simulink model "EKF_sim"  (R2020a)
settings: Solver=VariableStepAuto  StartTime=0.0  StopTime=694  RelTol=1e-3
values from neighbouring files (symbols this model uses):
  acc_variance = 4.8e-1    (= 0.48)    [init.m]
  bias_acc_variance = 4e-10    [init.m]
  bias_gyro_variance = 4e-14    [init.m]
  DT = EKF_DT    (= 0.02)    [init.m]
  EKF_DT = 0.02    [init.m]
  g = 9.81    [init.m]
  GPS_variance = 1e-2    (= 0.01)    [init.m]
  gyro_variance = 4.8e-2    (= 0.048)    [init.m]
  head_variance = 7e-3    (= 0.007)    [init.m]
  init_time = 11    [init.m]
  lambda_xa = 1e-4    (= 0.0001)    [init.m]
  lambda_xg = 1e-3    (= 0.001)    [init.m]
  SHOE_buffer_N = 100    [init.m]
  SHOE_threshold = 30    [init.m]
  t1_end = 291    [init.m]
  t1_start = 290    [init.m]
  t2_end = 392.5    [init.m]
  t2_start = 392    [init.m]
  t3_end = 420    [init.m]
  t3_start = 419    [init.m]
  t4_end = 439    [init.m]
  t4_start = 438    [init.m]
  vel_variance = 1e-2    (= 0.01)    [init.m]
  zero_vel_period = 50000    [init.m]
(part 4 of 5)

== matlab function EKF_sim/EKF_bias/System Prediction/prediction_step ==
  data: x0 input; x_k output; P0 input; x_k_1 input size=22 1; P_k_1 input size=22 22; yg input; ya input; lambda_xa parameter; lambda_xg parameter; U input; P_k output size=22 22; DT parameter; g parameter; flag_init input; flag_init_ output
% --------------------         prediction           -------------------- %
%{
% This function computes the prediction step of the Kalman Filter. After 
% the initialization of the system, at each period the state vector is 
% updated, related to the prediction function and the measurement by the 
% inertial sensors (gyroscope and accelerometer). The covariance matrix P 
% is also updated.

% Input:
%     x0         : initial vector state
%     P0         : initial matrix P
%     x_k_1      : state vector before prediction step
%     P_k_1      : matrix P before prediction step
%     yg         : gyroscope measurement
%     ya         : accelerometer measurement
%     lambda_xa  : correlation time of Accelerometer Bias
%     lambda_xg  : correlation time of Gyroscope Bias
%     U          : covariance Matrix of input sensor
%     DT         : period of EKF system
%     g          : gravity acceleration
%     flag_init  : flag for initialization task

% Output:
%     x_k        : state vector after prediction step
%     P_k        : matrix P after prediction step
%     flag_init_ : flag for initialization task

% State vector x = [q w xg r v a xa]' [22x1]:
% q  = [q1 q2 q3 q4]     unit quaternion representing the attitude (1 2 3 4)
% w  = [wx wy wz]        angular velocity (5 6 7)
% xg = [xg_x xg_y xg_z]  gyro bias (8 9 10)
% r  = [rx ry rz]        position (NED)(11 12 13)
% v  = [vx vy vz]        linear velocity (NED) (14 15 16)
% a  = [ax ay az]        linear acceleration (NED) (17 18 19)
% xa = [xa_x xa_y xa_z]  accelerometer bias (20 21 22)
 
% Prediction model functions:
% fq = q * q(w*DT)
% fw = (yg-xg);
% fxg = (1-lambda_xg*DT)*xg+vxg;
% fr = r + v*DT + a*DT*DT/2;
% fv = v + a*DT;
% fa = Rnb*(ya - xa) + [0;0;g];
% fxa = (1-lambda_xa*DT)*xa+vxa;

% P_k = Fx*P_k_1*Fx' + Fu*U*Fu'
 
% U = [gyro_variance(3x3),       0               0               0
%        0           bias_gyro_variance(3x3)     0               0
%        0                       0        acc_variance(3x3)      0
%        0                       0                  bias_acc_variance(3x3)]

% See 'calcolo_matrice_F.m' for the exact calculation of matrices Fx and Fu
% These matrices are calculated offline, so note that if same parameters of 
% the system change, these matrices need to be changed.
%}
%%
function [x_k,  P_k, flag_init_] = prediction(x0, P0, x_k_1, P_k_1, ...
                                          yg, ya, lambda_xa, lambda_xg,...
                                          U, DT, g, flag_init)
    x_k = zeros(22,1);
    P_k = zeros(22,22);
    flag_init_ = flag_init;
    if flag_init ~= 0           %initialization check
        if flag_init == 1
            x_k_1 = x0;
            P_k_1 = P0;
            flag_init_ = 2;     %set flag=2 so the initialization is done
        end                     %one time only
        
        % Prediction Step
        [q_k_1,~,xg_k_1,r_k_1,v_k_1,~,xa_k_1] = extract_var(x_k_1);
        
        xg_k = (1 - lambda_xg*DT)*xg_k_1;               %Gyro's Bias update
        w_k  = (yg - xg_k_1);                           %Velocity Rotation update
        w_DT = (w_k*DT);                                %Angular displacement in DT time interval
        q_w  = new_q(w_DT(1),w_DT(2),w_DT(3));                        
        q    = q_product(q_k_1,q_w);                    %Rotations composition
        norm = (q(1)^2 + q(2)^2 + q(3)^2 + q(4)^2)^0.5;
        q_k  = q/norm;                                  %Normalize new quaternion
        Rnb  = fromq2rot(q_k(1),q_k(2),q_k(3),q_k(4));
       
        xa_k = (1-lambda_xa*DT)*xa_k_1;                 %Accelerometer's Bias update
        a_k  = Rnb*(ya-xa_k_1) + [0;0;g];               %Acceleration Update
        v_k  = v_k_1 + a_k*DT;                          %Velocity update
        r_k  = r_k_1 + v_k*DT + a_k*DT*DT/2;            %Position update (origin of body frame)
        
        x_k = compact_var(q_k, w_k,  xg_k, r_k, v_k, a_k, xa_k);          
        
        Fu = calcolo_Fu(q_k(1),q_k(2),q_k(3),q_k(4));
        Fx = calcolo_Fx(q_k(1),q_k(2),q_k(3),q_k(4),w_k(1),w_k(2),w_k(3),ya(1),ya(2),ya(3),xa_k(1),xa_k(2),xa_k(3));
        P_k = Fx*P_k_1*Fx' + Fu*U*Fu';                  %Matrix P Update           
    end
end

%% Auxiliary Functions
% This function extracts single variables from the state vector
function [q, w,  xg, r, v, a, xa] = extract_var(x)
    q  = x(1:4);
    w  = x(5:7);
    xg = x(8:10);
    r  = x(11:13);
    v  = x(14:16);
    a  = x(17:19);
    xa = x(20:22);
end

% This function compacts single variables into the state vector
function x = compact_var(q, w,  xg, r, v, a, xa)
    x = zeros(22,1);
    x(1:4)   = q;
    x(5:7)   = w;
    x(8:10)  = xg;
    x(11:13) = r;
    x(14:16) = v;
    x(17:19) = a;
    x(20:22) = xa;
end

% This function computes the body-to-nav rotation matrix from quaternion
function rot = fromq2rot(q1,q2,q3,q4)
    rot = [q1^2+q2^2-q3^2-q4^2, 2*(q2*q3-q1*q4), 2*(q1*q3+q2*q4); ...
           2*(q2*q3+q1*q4), q1^2-q2^2+q3^2-q4^2, 2*(q3*q4-q1*q2); ...
           2*(q2*q4-q1*q3), 2*(q1*q2+q3*q4), q1^2-q2^2-q3^2+q4^2];
end

% This function create a quaternion from Euler's angle [Yaw,Pitch,Roll]
function q = new_q(yaw,pitch,roll)
    q = zeros(1,4);
    q(1) = cos(roll/2) * cos(pitch/2) * cos(yaw/2) + sin(roll/2) * sin(pitch/2) * sin(yaw/2);
    q(2) = sin(roll/2) * cos(pitch/2) * cos(yaw/2) - cos(roll/2) * sin(pitch/2) * sin(yaw/2);
    q(3) = cos(roll/2) * sin(pitch/2) * cos(yaw/2) + sin(roll/2) * cos(pitch/2) * sin(yaw/2);
    q(4) = cos(roll/2) * cos(pitch/2) * sin(yaw/2) - sin(roll/2) * sin(pitch/2) * cos(yaw/2);
    
end

% This function computes the product between two quaternion
function q = q_product(a,b)
    q = zeros(1,4);
    q(1) = b(1)*a(1) - b(2)*a(2) - b(3)*a(3) - b(4)*a(4);
    q(2) = b(1)*a(2) + b(2)*a(1) - b(3)*a(4) + b(4)*a(3);
    q(3) = b(1)*a(3) + b(2)*a(4) + b(3)*a(1) - b(4)*a(2);
    q(4) = b(1)*a(4) - b(2)*a(3) + b(3)*a(2) + b(4)*a(1);
end
%%
% These functions calculate the Fx and Fu matrices. 
% See 'calcolo_matrice_F.m' for the symbolic calculation used
function Fx = calcolo_Fx(q1,q2,q3,q4,w_yaw,w_pitch,w_roll,ya1,ya2,ya3,xa_x,xa_y,xa_z)
Fx =[(cos(w_pitch/100)*cos(w_roll/100)*cos(w_yaw/100) + sin(w_pitch/100)*sin(w_roll/100)*sin(w_yaw/100))/(q1^2 + q2^2 + q3^2 + q4^2)^(1/2) + (q1*(q2*(cos(w_pitch/100)*cos(w_yaw/100)*sin(w_roll/100) - cos(w_roll/100)*sin(w_pitch/100)*sin(w_yaw/100)) - q1*(cos(w_pitch/100)*cos(w_roll/100)*cos(w_yaw/100) + sin(w_pitch/100)*sin(w_roll/100)*sin(w_yaw/100)) + q3*(cos(w_roll/100)*cos(w_yaw/100)*sin(w_pitch/100) + cos(w_pitch/100)*sin(w_roll/100)*sin(w_yaw/100)) + q4*(cos(w_pitch/100)*cos(w_roll/100)*sin(w_yaw/100) - cos(w_yaw/100)*sin(w_pitch/100)*sin(w_roll/100))))/(q1^2 + q2^2 + q3^2 + q4^2)^(3/2),   (q2*(q2*(cos(w_pitch/100)*cos(w_yaw/100)*sin(w_roll/100) - cos(w_roll/100)*sin(w_pitch/100)*sin(w_yaw/100)) - q1*(cos(w_pitch/100)*cos(w_roll/100)*cos(w_yaw/100) + sin(w_pitch/100)*sin(w_roll/100)*sin(w_yaw/100)) + q3*(cos(w_roll/100)*cos(w_yaw/100)*sin(w_pitch/100) + cos(w_pitch/100)*sin(w_roll/100)*sin(w_yaw/100)) + q4*(cos(w_pitch/100)*cos(w_roll/100)*sin(w_yaw/100) - cos(w_yaw/100)*sin(w_pitch/100)*sin(w_roll/100))))/(q1^2 + q2^2 + q3^2 + q4^2)^(3/2) - (cos(w_pitch/100)*cos(w_yaw/100)*sin(w_roll/100) - cos(w_roll/100)*sin(w_pitch/100)*sin(w_yaw/100))/(q1^2 + q2^2 + q3^2 + q4^2)^(1/2),   (q3*(q2*(cos(w_pitch/100)*cos(w_yaw/100)*sin(w_roll/100) - cos(w_roll/100)*sin(w_pitch/100)*sin(w_yaw/100)) - q1*(cos(w_pitch/100)*cos(w_roll/100)*cos(w_yaw/100) + sin(w_pitch/100)*sin(w_roll/100)*sin(w_yaw/100)) + q3*(cos(w_roll/100)*cos(w_yaw/100)*sin(w_pitch/100) + cos(w_pitch/100)*sin(w_roll/100)*sin(w_yaw/100)) + q4*(cos(w_pitch/100)*cos(w_roll/100)*sin(w_yaw/100) - cos(w_yaw/100)*sin(w_pitch/100)*sin(w_roll/100))))/(q1^2 + q2^2 + q3^2 + q4^2)^(3/2) - (cos(w_roll/100)*cos(w_yaw/100)*sin(w_pitch/100) + cos(w_pitch/100)*sin(w_roll/100)*sin(w_yaw/100))/(q1^2 + q2^2 + q3^2 + q4^2)^(1/2),   (q4*(q2*(cos(w_pitch/100)*cos(w_yaw/100)*sin(w_roll/100) - cos(w_roll/100)*sin(w_pitch/100)*sin(w_yaw/100)) - q1*(cos(w_pitch/100)*cos(w_roll/100)*cos(w_yaw/100) + sin(w_pitch/100)*sin(w_roll/100)*sin(w_yaw/100)) + q3*(cos(w_roll/100)*cos(w_yaw/100)*sin(w_pitch/100) + cos(w_pitch/100)*sin(w_roll/100)*sin(w_yaw/100)) + q4*(cos(w_pitch/100)*cos(w_roll/100)*sin(w_yaw/100) - cos(w_yaw/100)*sin(w_pitch/100)*sin(w_roll/100))))/(q1^2 + q2^2 + q3^2 + q4^2)^(3/2) - (cos(w_pitch/100)*cos(w_roll/100)*sin(w_yaw/100) - cos(w_yaw/100)*sin(w_pitch/100)*sin(w_roll/100))/(q1^2 + q2^2 + q3^2 + q4^2)^(1/2), -(q1*((cos(w_pitch/100)*cos(w_roll/100)*sin(w_yaw/100))/100 - (cos(w_yaw/100)*sin(w_pitch/100)*sin(w_roll/100))/100) - q2*((cos(w_roll/100)*cos(w_yaw/100)*sin(w_pitch/100))/100 + (cos(w_pitch/100)*sin(w_roll/100)*sin(w_yaw/100))/100) + q3*((cos(w_pitch/100)*cos(w_yaw/100)*sin(w_roll/100))/100 - (cos(w_roll/100)*sin(w_pitch/100)*sin(w_yaw/100))/100) + q4*((cos(w_pitch/100)*cos(w_roll/100)*cos(w_yaw/100))/100 + (sin(w_pitch/100)*sin(w_roll/100)*sin(w_yaw/100))/100))/(q1^2 + q2^2 + q3^2 + q4^2)^(1/2), -(q1*((cos(w_roll/100)*cos(w_yaw/100)*sin(w_pitch/100))/100 - (cos(w_pitch/100)*sin(w_roll/100)*sin(w_yaw/100))/100) - q2*((cos(w_pitch/100)*cos(w_roll/100)*sin(w_yaw/100))/100 + (cos(w_yaw/100)*sin(w_pitch/100)*sin(w_roll/100))/100) + q3*((cos(w_pitch/100)*cos(w_roll/100)*cos(w_yaw/100))/100 - (sin(w_pitch/100)*sin(w_roll/100)*sin(w_yaw/100))/100) - q4*((cos(w_pitch/100)*cos(w_yaw/100)*sin(w_roll/100))/100 + (cos(w_roll/100)*sin(w_pitch/100)*sin(w_yaw/100))/100))/(q1^2 + q2^2 + q3^2 + q4^2)^(1/2), -(q1*((cos(w_pitch/100)*cos(w_yaw/100)*sin(w_roll/100))/100 - (cos(w_roll/100)*sin(w_pitch/100)*sin(w_yaw/100))/100) + q2*((cos(w_pitch/100)*cos(w_roll/100)*cos(w_yaw/100))/100 + (sin(w_pitch/100)*sin(w_roll/100)*sin(w_yaw/100))/100) + q3*((cos(w_pitch/100)*cos(w_roll/100)*sin(w_yaw/100))/100 - (cos(w_yaw/100)*sin(w_pitch/100)*sin(w_roll/100))/100) - q4*((cos(w_roll/100)*cos(w_yaw/100)*sin(w_pitch/100))/100 + (cos(w_pitch/100)*sin(w_roll/100)*sin(w_yaw/100))/100))/(q1^2 + q2^2 + q3^2 + q4^2)^(1/2),           0,           0,           0, 0, 0, 0,    0,    0,    0,      0,      0,      0,                                 0,                                 0,                                 0;
     (cos(w_pitch/100)*cos(w_yaw/100)*sin(w_roll/100) - cos(w_roll/100)*sin(w_pitch/100)*sin(w_yaw/100))/(q1^2 + q2^2 + q3^2 + q4^2)^(1/2) - (q1*(q1*(cos(w_pitch/100)*cos(w_yaw/100)*sin(w_roll/100) - cos(w_roll/100)*sin(w_pitch/100)*sin(w_yaw/100)) + q2*(cos(w_pitch/100)*cos(w_roll/100)*cos(w_yaw/100) + sin(w_pitch/100)*sin(w_roll/100)*sin(w_yaw/100)) + q3*(cos(w_pitch/100)*cos(w_roll/100)*sin(w_yaw/100) - cos(w_yaw/100)*sin(w_pitch/100)*sin(w_roll/100)) - q4*(cos(w_roll/100)*cos(w_yaw/100)*sin(w_pitch/100) + cos(w_pitch/100)*sin(w_roll/100)*sin(w_yaw/100))))/(q1^2 + q2^2 + q3^2 + q4^2)^(3/2),   (cos(w_pitch/100)*cos(w_roll/100)*cos(w_yaw/100) + sin(w_pitch/100)*sin(w_roll/100)*sin(w_yaw/100))/(q1^2 + q2^2 + q3^2 + q4^2)^(1/2) - (q2*(q1*(cos(w_pitch/100)*cos(w_yaw/100)*sin(w_roll/100) - cos(w_roll/100)*sin(w_pitch/100)*sin(w_yaw/100)) + q2*(cos(w_pitch/100)*cos(w_roll/100)*cos(w_yaw/100) + sin(w_pitch/100)*sin(w_roll/100)*sin(w_yaw/100)) + q3*(cos(w_pitch/100)*cos(w_roll/100)*sin(w_yaw/100) - cos(w_yaw/100)*sin(w_pitch/100)*sin(w_roll/100)) - q4*(cos(w_roll/100)*cos(w_yaw/100)*sin(w_pitch/100) + cos(w_pitch/100)*sin(w_roll/100)*sin(w_yaw/100))))/(q1^2 + q2^2 + q3^2 + q4^2)^(3/2),   (cos(w_pitch/100)*cos(w_roll/100)*sin(w_yaw/100) - cos(w_yaw/100)*sin(w_pitch/100)*sin(w_roll/100))/(q1^2 + q2^2 + q3^2 + q4^2)^(1/2) - (q3*(q1*(cos(w_pitch/100)*cos(w_yaw/100)*sin(w_roll/100) - cos(w_roll/100)*sin(w_pitch/100)*sin(w_yaw/100)) + q2*(cos(w_pitch/100)*cos(w_roll/100)*cos(w_yaw/100) + sin(w_pitch/100)*sin(w_roll/100)*sin(w_yaw/100)) + q3*(cos(w_pitch/100)*cos(w_roll/100)*sin(w_yaw/100) - cos(w_yaw/100)*sin(w_pitch/100)*sin(w_roll/100)) - q4*(cos(w_roll/100)*cos(w_yaw/100)*sin(w_pitch/100) + cos(w_pitch/100)*sin(w_roll/100)*sin(w_yaw/100))))/(q1^2 + q2^2 + q3^2 + q4^2)^(3/2), - (cos(w_roll/100)*cos(w_yaw/100)*sin(w_pitch/100) + cos(w_pitch/100)*sin(w_roll/100)*sin(w_yaw/100))/(q1^2 + q2^2 + q3^2 + q4^2)^(1/2) - (q4*(q1*(cos(w_pitch/100)*cos(w_yaw/100)*sin(w_roll/100) - cos(w_roll/100)*sin(w_pitch/100)*sin(w_yaw/100)) + q2*(cos(w_pitch/100)*cos(w_roll/100)*cos(w_yaw/100) + sin(w_pitch/100)*sin(w_roll/100)*sin(w_yaw/100)) + q3*(cos(w_pitch/100)*cos(w_roll/100)*sin(w_yaw/100) - cos(w_yaw/100)*sin(w_pitch/100)*sin(w_roll/100)) - q4*(cos(w_roll/100)*cos(w_yaw/100)*sin(w_pitch/100) + cos(w_pitch/100)*sin(w_roll/100)*sin(w_yaw/100))))/(q1^2 + q2^2 + q3^2 + q4^2)^(3/2), -(q1*((cos(w_roll/100)*cos(w_yaw/100)*sin(w_pitch/100))/100 + (cos(w_pitch/100)*sin(w_roll/100)*sin(w_yaw/100))/100) + q2*((cos(w_pitch/100)*cos(w_roll/100)*sin(w_yaw/100))/100 - (cos(w_yaw/100)*sin(w_pitch/100)*sin(w_roll/100))/100) - q3*((cos(w_pitch/100)*cos(w_roll/100)*cos(w_yaw/100))/100 + (sin(w_pitch/100)*sin(w_roll/100)*sin(w_yaw/100))/100) + q4*((cos(w_pitch/100)*cos(w_yaw/100)*sin(w_roll/100))/100 - (cos(w_roll/100)*sin(w_pitch/100)*sin(w_yaw/100))/100))/(q1^2 + q2^2 + q3^2 + q4^2)^(1/2), -(q1*((cos(w_pitch/100)*cos(w_roll/100)*sin(w_yaw/100))/100 + (cos(w_yaw/100)*sin(w_pitch/100)*sin(w_roll/100))/100) + q2*((cos(w_roll/100)*cos(w_yaw/100)*sin(w_pitch/100))/100 - (cos(w_pitch/100)*sin(w_roll/100)*sin(w_yaw/100))/100) + q3*((cos(w_pitch/100)*cos(w_yaw/100)*sin(w_roll/100))/100 + (cos(w_roll/100)*sin(w_pitch/100)*sin(w_yaw/100))/100) + q4*((cos(w_pitch/100)*cos(w_roll/100)*cos(w_yaw/100))/100 - (sin(w_pitch/100)*sin(w_roll/100)*sin(w_yaw/100))/100))/(q1^2 + q2^2 + q3^2 + q4^2)^(1/2), -(q2*((cos(w_pitch/100)*cos(w_yaw/100)*sin(w_roll/100))/100 - (cos(w_roll/100)*sin(w_pitch/100)*sin(w_yaw/100))/100) - q1*((cos(w_pitch/100)*cos(w_roll/100)*cos(w_yaw/100))/100 + (sin(w_pitch/100)*sin(w_roll/100)*sin(w_yaw/100))/100) + q3*((cos(w_roll/100)*cos(w_yaw/100)*sin(w_pitch/100))/100 + (cos(w_pitch/100)*sin(w_roll/100)*sin(w_yaw/100))/100) + q4*((cos(w_pitch/100)*cos(w_roll/100)*sin(w_yaw/100))/100 - (cos(w_yaw/100)*sin(w_pitch/100)*sin(w_roll/100))/100))/(q1^2 + q2^2 + q3^2 + q4^2)^(1/2),           0,           0,           0, 0, 0, 0,    0,    0,    0,      0,      0,      0,                                 0,                                 0,                                 0;
     (cos(w_roll/100)*cos(w_yaw/100)*sin(w_pitch/100) + cos(w_pitch/100)*sin(w_roll/100)*sin(w_yaw/100))/(q1^2 + q2^2 + q3^2 + q4^2)^(1/2) - (q1*(q1*(cos(w_roll/100)*cos(w_yaw/100)*sin(w_pitch/100) + cos(w_pitch/100)*sin(w_roll/100)*sin(w_yaw/100)) - q2*(cos(w_pitch/100)*cos(w_roll/100)*sin(w_yaw/100) - cos(w_yaw/100)*sin(w_pitch/100)*sin(w_roll/100)) + q3*(cos(w_pitch/100)*cos(w_roll/100)*cos(w_yaw/100) + sin(w_pitch/100)*sin(w_roll/100)*sin(w_yaw/100)) + q4*(cos(w_pitch/100)*cos(w_yaw/100)*sin(w_roll/100) - cos(w_roll/100)*sin(w_pitch/100)*sin(w_yaw/100))))/(q1^2 + q2^2 + q3^2 + q4^2)^(3/2), - (cos(w_pitch/100)*cos(w_roll/100)*sin(w_yaw/100) - cos(w_yaw/100)*sin(w_pitch/100)*sin(w_roll/100))/(q1^2 + q2^2 + q3^2 + q4^2)^(1/2) - (q2*(q1*(cos(w_roll/100)*cos(w_yaw/100)*sin(w_pitch/100) + cos(w_pitch/100)*sin(w_roll/100)*sin(w_yaw/100)) - q2*(cos(w_pitch/100)*cos(w_roll/100)*sin(w_yaw/100) - cos(w_yaw/100)*sin(w_pitch/100)*sin(w_roll/100)) + q3*(cos(w_pitch/100)*cos(w_roll/100)*cos(w_yaw/100) + sin(w_pitch/100)*sin(w_roll/100)*sin(w_yaw/100)) + q4*(cos(w_pitch/100)*cos(w_yaw/100)*sin(w_roll/100) - cos(w_roll/100)*sin(w_pitch/100)*sin(w_yaw/100))))/(q1^2 + q2^2 + q3^2 + q4^2)^(3/2),   (cos(w_pitch/100)*cos(w_roll/100)*cos(w_yaw/100) + sin(w_pitch/100)*sin(w_roll/100)*sin(w_yaw/100))/(q1^2 + q2^2 + q3^2 + q4^2)^(1/2) - (q3*(q1*(cos(w_roll/100)*cos(w_yaw/100)*sin(w_pitch/100) + cos(w_pitch/100)*sin(w_roll/100)*sin(w_yaw/100)) - q2*(cos(w_pitch/100)*cos(w_roll/100)*sin(w_yaw/100) - cos(w_yaw/100)*sin(w_pitch/100)*sin(w_roll/100)) + q3*(cos(w_pitch/100)*cos(w_roll/100)*cos(w_yaw/100) + sin(w_pitch/100)*sin(w_roll/100)*sin(w_yaw/100)) + q4*(cos(w_pitch/100)*cos(w_yaw/100)*sin(w_roll/100) - cos(w_roll/100)*sin(w_pitch/100)*sin(w_yaw/100))))/(q1^2 + q2^2 + q3^2 + q4^2)^(3/2),   (cos(w_pitch/100)*cos(w_yaw/100)*sin(w_roll/100) - cos(w_roll/100)*sin(w_pitch/100)*sin(w_yaw/100))/(q1^2 + q2^2 + q3^2 + q4^2)^(1/2) - (q4*(q1*(cos(w_roll/100)*cos(w_yaw/100)*sin(w_pitch/100) + cos(w_pitch/100)*sin(w_roll/100)*sin(w_yaw/100)) - q2*(cos(w_pitch/100)*cos(w_roll/100)*sin(w_yaw/100) - cos(w_yaw/100)*sin(w_pitch/100)*sin(w_roll/100)) + q3*(cos(w_pitch/100)*cos(w_roll/100)*cos(w_yaw/100) + sin(w_pitch/100)*sin(w_roll/100)*sin(w_yaw/100)) + q4*(cos(w_pitch/100)*cos(w_yaw/100)*sin(w_roll/100) - cos(w_roll/100)*sin(w_pitch/100)*sin(w_yaw/100))))/(q1^2 + q2^2 + q3^2 + q4^2)^(3/2), -(q2*((cos(w_pitch/100)*cos(w_roll/100)*cos(w_yaw/100))/100 + (sin(w_pitch/100)*sin(w_roll/100)*sin(w_yaw/100))/100) - q1*((cos(w_pitch/100)*cos(w_yaw/100)*sin(w_roll/100))/100 - (cos(w_roll/100)*sin(w_pitch/100)*sin(w_yaw/100))/100) + q3*((cos(w_pitch/100)*cos(w_roll/100)*sin(w_yaw/100))/100 - (cos(w_yaw/100)*sin(w_pitch/100)*sin(w_roll/100))/100) + q4*((cos(w_roll/100)*cos(w_yaw/100)*sin(w_pitch/100))/100 + (cos(w_pitch/100)*sin(w_roll/100)*sin(w_yaw/100))/100))/(q1^2 + q2^2 + q3^2 + q4^2)^(1/2),  (q1*((cos(w_pitch/100)*cos(w_roll/100)*cos(w_yaw/100))/100 - (sin(w_pitch/100)*sin(w_roll/100)*sin(w_yaw/100))/100) + q2*((cos(w_pitch/100)*cos(w_yaw/100)*sin(w_roll/100))/100 + (cos(w_roll/100)*sin(w_pitch/100)*sin(w_yaw/100))/100) - q3*((cos(w_roll/100)*cos(w_yaw/100)*sin(w_pitch/100))/100 - (cos(w_pitch/100)*sin(w_roll/100)*sin(w_yaw/100))/100) - q4*((cos(w_pitch/100)*cos(w_roll/100)*sin(w_yaw/100))/100 + (cos(w_yaw/100)*sin(w_pitch/100)*sin(w_roll/100))/100))/(q1^2 + q2^2 + q3^2 + q4^2)^(1/2),  (q1*((cos(w_pitch/100)*cos(w_roll/100)*sin(w_yaw/100))/100 - (cos(w_yaw/100)*sin(w_pitch/100)*sin(w_roll/100))/100) + q2*((cos(w_roll/100)*cos(w_yaw/100)*sin(w_pitch/100))/100 + (cos(w_pitch/100)*sin(w_roll/100)*sin(w_yaw/100))/100) - q3*((cos(w_pitch/100)*cos(w_yaw/100)*sin(w_roll/100))/100 - (cos(w_roll/100)*sin(w_pitch/100)*sin(w_yaw/100))/100) + q4*((cos(w_pitch/100)*cos(w_roll/100)*cos(w_yaw/100))/100 + (sin(w_pitch/100)*sin(w_roll/100)*sin(w_yaw/100))/100))/(q1^2 + q2^2 + q3^2 + q4^2)^(1/2),           0,           0,           0, 0, 0, 0,    0,    0,    0,      0,      0,      0,                                 0,                                 0,                                 0;
     (cos(w_pitch/100)*cos(w_roll/100)*sin(w_yaw/100) - cos(w_yaw/100)*sin(w_pitch/100)*sin(w_roll/100))/(q1^2 + q2^2 + q3^2 + q4^2)^(1/2) - (q1*(q1*(cos(w_pitch/100)*cos(w_roll/100)*sin(w_yaw/100) - cos(w_yaw/100)*sin(w_pitch/100)*sin(w_roll/100)) + q2*(cos(w_roll/100)*cos(w_yaw/100)*sin(w_pitch/100) + cos(w_pitch/100)*sin(w_roll/100)*sin(w_yaw/100)) - q3*(cos(w_pitch/100)*cos(w_yaw/100)*sin(w_roll/100) - cos(w_roll/100)*sin(w_pitch/100)*sin(w_yaw/100)) + q4*(cos(w_pitch/100)*cos(w_roll/100)*cos(w_yaw/100) + sin(w_pitch/100)*sin(w_roll/100)*sin(w_yaw/100))))/(q1^2 + q2^2 + q3^2 + q4^2)^(3/2),   (cos(w_roll/100)*cos(w_yaw/100)*sin(w_pitch/100) + cos(w_pitch/100)*sin(w_roll/100)*sin(w_yaw/100))/(q1^2 + q2^2 + q3^2 + q4^2)^(1/2) - (q2*(q1*(cos(w_pitch/100)*cos(w_roll/100)*sin(w_yaw/100) - cos(w_yaw/100)*sin(w_pitch/100)*sin(w_roll/100)) + q2*(cos(w_roll/100)*cos(w_yaw/100)*sin(w_pitch/100) + cos(w_pitch/100)*sin(w_roll/100)*sin(w_yaw/100)) - q3*(cos(w_pitch/100)*cos(w_yaw/100)*sin(w_roll/100) - cos(w_roll/100)*sin(w_pitch/100)*sin(w_yaw/100)) + q4*(cos(w_pitch/100)*cos(w_roll/100)*cos(w_yaw/100) + sin(w_pitch/100)*sin(w_roll/100)*sin(w_yaw/100))))/(q1^2 + q2^2 + q3^2 + q4^2)^(3/2), - (cos(w_pitch/100)*cos(w_yaw/100)*sin(w_roll/100) - cos(w_roll/100)*sin(w_pitch/100)*sin(w_yaw/100))/(q1^2 + q2^2 + q3^2 + q4^2)^(1/2) - (q3*(q1*(cos(w_pitch/100)*cos(w_roll/100)*sin(w_yaw/100) - cos(w_yaw/100)*sin(w_pitch/100)*sin(w_roll/100)) + q2*(cos(w_roll/100)*cos(w_yaw/100)*sin(w_pitch/100) + cos(w_pitch/100)*sin(w_roll/100)*sin(w_yaw/100)) - q3*(cos(w_pitch/100)*cos(w_yaw/100)*sin(w_roll/100) - cos(w_roll/100)*sin(w_pitch/100)*sin(w_yaw/100)) + q4*(cos(w_pitch/100)*cos(w_roll/100)*cos(w_yaw/100) + sin(w_pitch/100)*sin(w_roll/100)*sin(w_yaw/100))))/(q1^2 + q2^2 + q3^2 + q4^2)^(3/2),   (cos(w_pitch/100)*cos(w_roll/100)*cos(w_yaw/100) + sin(w_pitch/100)*sin(w_roll/100)*sin(w_yaw/100))/(q1^2 + q2^2 + q3^2 + q4^2)^(1/2) - (q4*(q1*(cos(w_pitch/100)*cos(w_roll/100)*sin(w_yaw/100) - cos(w_yaw/100)*sin(w_pitch/100)*sin(w_roll/100)) + q2*(cos(w_roll/100)*cos(w_yaw/100)*sin(w_pitch/100) + cos(w_pitch/100)*sin(w_roll/100)*sin(w_yaw/100)) - q3*(cos(w_pitch/100)*cos(w_yaw/100)*sin(w_roll/100) - cos(w_roll/100)*sin(w_pitch/100)*sin(w_yaw/100)) + q4*(cos(w_pitch/100)*cos(w_roll/100)*cos(w_yaw/100) + sin(w_pitch/100)*sin(w_roll/100)*sin(w_yaw/100))))/(q1^2 + q2^2 + q3^2 + q4^2)^(3/2),  (q1*((cos(w_pitch/100)*cos(w_roll/100)*cos(w_yaw/100))/100 + (sin(w_pitch/100)*sin(w_roll/100)*sin(w_yaw/100))/100) + q2*((cos(w_pitch/100)*cos(w_yaw/100)*sin(w_roll/100))/100 - (cos(w_roll/100)*sin(w_pitch/100)*sin(w_yaw/100))/100) + q3*((cos(w_roll/100)*cos(w_yaw/100)*sin(w_pitch/100))/100 + (cos(w_pitch/100)*sin(w_roll/100)*sin(w_yaw/100))/100) - q4*((cos(w_pitch/100)*cos(w_roll/100)*sin(w_yaw/100))/100 - (cos(w_yaw/100)*sin(w_pitch/100)*sin(w_roll/100))/100))/(q1^2 + q2^2 + q3^2 + q4^2)^(1/2), -(q1*((cos(w_pitch/100)*cos(w_yaw/100)*sin(w_roll/100))/100 + (cos(w_roll/100)*sin(w_pitch/100)*sin(w_yaw/100))/100) - q2*((cos(w_pitch/100)*cos(w_roll/100)*cos(w_yaw/100))/100 - (sin(w_pitch/100)*sin(w_roll/100)*sin(w_yaw/100))/100) - q3*((cos(w_pitch/100)*cos(w_roll/100)*sin(w_yaw/100))/100 + (cos(w_yaw/100)*sin(w_pitch/100)*sin(w_roll/100))/100) + q4*((cos(w_roll/100)*cos(w_yaw/100)*sin(w_pitch/100))/100 - (cos(w_pitch/100)*sin(w_roll/100)*sin(w_yaw/100))/100))/(q1^2 + q2^2 + q3^2 + q4^2)^(1/2), -(q1*((cos(w_roll/100)*cos(w_yaw/100)*sin(w_pitch/100))/100 + (cos(w_pitch/100)*sin(w_roll/100)*sin(w_yaw/100))/100) - q2*((cos(w_pitch/100)*cos(w_roll/100)*sin(w_yaw/100))/100 - (cos(w_yaw/100)*sin(w_pitch/100)*sin(w_roll/100))/100) + q3*((cos(w_pitch/100)*cos(w_roll/100)*cos(w_yaw/100))/100 + (sin(w_pitch/100)*sin(w_roll/100)*sin(w_yaw/100))/100) + q4*((cos(w_pitch/100)*cos(w_yaw/100)*sin(w_roll/100))/100 - (cos(w_roll/100)*sin(w_pitch/100)*sin(w_yaw/100))/100))/(q1^2 + q2^2 + q3^2 + q4^2)^(1/2),           0,           0,           0, 0, 0, 0,    0,    0,    0,      0,      0,      0,                                 0,                                 0,                                 0;
                                                                                                                                                                                                                                                                                                                                                                                                                                                                                                                                                                                                                      0,                                                                                                                                                                                                                                                                                                                                                                                                                                                                                                                                                                                                                    0,                                                                                                                                                                                                                                                                                                                                                                                                                                                                                                                                                                                                                    0,                                                                                                                                                                                                                                                                                                                                                                                                                                                                                                                                                                                                                    0,                                                                                                                                                                                                                                                                                                                                                                                                                                                                                                                      0,                                                                                                                                                                                                                                                                                                                                                                                                                                                                                                                      0,                                                                                                                                                                                                                                                                                                                                                                                                                                                                                                                      0,          -1,           0,           0, 0, 0, 0,    0,    0,    0,      0,      0,      0,                                 0,                                 0,                                 0;
                                                                                                                                                                                                                                                                                                                                                                                                                                                                                                                                                                                                                      0,                                                                                                                                                                                                                                                                                                                                                                                                                                                                                                                                                                                                                    0,                                                                                                                                                                                                                                                                                                                                                                                                                                                                                                                                                                                                                    0,                                                                                                                                                                                                                                                                                                                                                                                                                                                                                                                                                                                                                    0,                                                                                                                                                                                                                                                                                                                                                                                                                                                                                                                      0,                                                                                                                                                                                                                                                                                                                                                                                                                                                                                                                      0,                                                                                                                                                                                                                                                                                                                                                                                                                                                                                                                      0,           0,          -1,           0, 0, 0, 0,    0,    0,    0,      0,      0,      0,                                 0,                                 0,                                 0;
                                                                                                                                                                                                                                                                                                                                                                                                                                                                                                                                                                                                                      0,                                                                                                                                                                                                                                                                                                                                                                                                                                                                                                                                                                                                                    0,                                                                                                                                                                                                                                                                                                                                                                                                                                                                                                                                                                                                                    0,                                                                                                                                                                                                                                                                                                                                                                                                                                                                                                                                                                                                                    0,                                                                                                                                                                                                                                                                                                                                                                                                                                                                                                                      0,                                                                                                                                                                                                                                                                                                                                                                                                                                                                                                                      0,                                                                                                                                                                                                                                                                                                                                                                                                                                                                                                                      0,           0,           0,          -1, 0, 0, 0,    0,    0,    0,      0,      0,      0,                                 0,                                 0,                                 0;
                                                                                                                                                                                                                                                                                                                                                                                                                                                                                                                                                                                                                      0,                                                                                                                                                                                                                                                                                                                                                                                                                                                                                                                                                                                                                    0,                                                                                                                                                                                                                                                                                                                                                                                                                                                                                                                                                                                                                    0,                                                                                                                                                                                                                                                                                                                                                                                                                                                                                                                                                                                                                    0,                                                                                                                                                                                                                                                                                                                                                                                                                                                                                                                      0,                                                                                                                                                                                                                                                                                                                                                                                                                                                                                                                      0,                                                                                                                                                                                                                                                                                                                                                                                                                                                                                                                      0, 49999/50000,           0,           0, 0, 0, 0,    0,    0,    0,      0,      0,      0,                                 0,                                 0,                                 0;
                                                                                                                                                                                                                                                                                                                                                                                                                                                                                                                                                                                                                      0,                                                                                                                                                                                                                                                                                                                                                                                                                                                                                                                                                                                                                    0,                                                                                                                                                                                                                                                                                                                                                                                                                                                                                                                                                                                                                    0,                                                                                                                                                                                                                                                                                                                                                                                                                                                                                                                                                                                                                    0,                                                                                                                                                                                                                                                                                                                                                                                                                                                                                                                      0,                                                                                                                                                                                                                                                                                                                                                                                                                                                                                                                      0,                                                                                                                                                                                                                                                                                                                                                                                                                                                                                                                      0,           0, 49999/50000,           0, 0, 0, 0,    0,    0,    0,      0,      0,      0,                                 0,                                 0,                                 0;
                                                                                                                                                                                                                                                                                                                                                                                                                                                                                                                                                                                                                      0,                                                                                                                                                                                                                                                                                                                                                                                                                                                                                                                                                                                                                    0,                                                                                                                                                                                                                                                                                                                                                                                                                                                                                                                                                                                                                    0,                                                                                                                                                                                                                                                                                                                                                                                                                                                                                                                                                                                                                    0,                                                                                                                                                                                                                                                                                                                                                                                                                                                                                                                      0,                                                                                                                                                                                                                                                                                                                                                                                                                                                                                                                      0,                                                                                                                                                                                                                                                                                                                                                                                                                                                                                                                      0,           0,           0, 49999/50000, 0, 0, 0,    0,    0,    0,      0,      0,      0,                                 0,                                 0,                                 0;
                                                                                                                                                                                                                                                                                                                                                                                                                                                                                                                                                                                                                      0,                                                                                                                                                                                                                                                                                                                                                                                                                                                                                                                                                                                                                    0,                                                                                                                                                                                                                                                                                                                                                                                                                                                                                                                                                                                                                    0,                                                                                                                                                                                                                                                                                                                                                                                                                                                                                                                                                                                                                    0,                                                                                                                                                                                                                                                                                                                                                                                                                                                                                                                      0,                                                                                                                                                                                                                                                                                                                                                                                                                                                                                                                      0,                                                                                                                                                                                                                                                                                                                                                                                                                                                                                                                      0,           0,           0,           0, 1, 0, 0, 1/50,    0,    0, 1/5000,      0,      0,                                 0,                                 0,                                 0;
                                                                                                                                                                                                                                                                                                                                                                                                                                                                                                                                                                                                                      0,                                                                                                                                                                                                                                                                                                                                                                                                                                                                                                                                                                                                                    0,                                                                                                                                                                                                                                                                                                                                                                                                                                                                                                                                                                                                                    0,                                                                                                                                                                                                                                                                                                                                                                                                                                                                                                                                                                                                                    0,                                                                                                                                                                                                                                                                                                                                                                                                                                                                                                                      0,                                                                                                                                                                                                                                                                                                                                                                                                                                                                                                                      0,                                                                                                                                                                                                                                                                                                                                                                                                                                                                                                                      0,           0,           0,           0, 0, 1, 0,    0, 1/50,    0,      0, 1/5000,      0,                                 0,                                 0,                                 0;
                                                                                                                                                                                                                                                                                                                                                                                                                                                                                                                                                                                                                      0,                                                                                                                                                                                                                                                                                                                                                                                                                                                                                                                                                                                                                    0,                                                                                                                                                                                                                                                                                                                                                                                                                                                                                                                                                                                                                    0,                                                                                                                                                                                                                                                                                                                                                                                                                                                                                                                                                                                                                    0,                                                                                                                                                                                                                                                                                                                                                                                                                                                                                                                      0,                                                                                                                                                                                                                                                                                                                                                                                                                                                                                                                      0,                                                                                                                                                                                                                                                                                                                                                                                                                                                                                                                      0,           0,           0,           0, 0, 0, 1,    0,    0, 1/50,      0,      0, 1/5000,                                 0,                                 0,                                 0;
                                                                                                                                                                                                                                                                                                                                                                                                                                                                                                                                                                                                                      0,                                                                                                                                                                                                                                                                                                                                                                                                                                                                                                                                                                                                                    0,                                                                                                                                                                                                                                                                                                                                                                                                                                                                                                                                                                                                                    0,                                                                                                                                                                                                                                                                                                                                                                                                                                                                                                                                                                                                                    0,                                                                                                                                                                                                                                                                                                                                                                                                                                                                                                                      0,                                                                                                                                                                                                                                                                                                                                                                                                                                                                                                                      0,                                                                                                                                                                                                                                                                                                                                                                                                                                                                                                                      0,           0,           0,           0, 0, 0, 0,    1,    0,    0,   1/50,      0,      0,                                 0,                                 0,                                 0;
                                                                                                                                                                                                                                                                                                                                                                                                                                                                                                                                                                                                                      0,                                                                                                                                                                                                                                                                                                                                                                                                                                                                                                                                                                                                                    0,                                                                                                                                                                                                                                                                                                                                                                                                                                                                                                                                                                                                                    0,                                                                                                                                                                                                                                                                                                                                                                                                                                                                                                                                                                                                                    0,                                                                                                                                                                                                                                                                                                                                                                                                                                                                                                                      0,                                                                                                                                                                                                                                                                                                                                                                                                                                                                                                                      0,                                                                                                                                                                                                                                                                                                                                                                                                                                                                                                                      0,           0,           0,           0, 0, 0, 0,    0,    1,    0,      0,   1/50,      0,                                 0,                                 0,                                 0;
                                                                                                                                                                                                                                                                                                                                                                                                                                                                                                                                                                                                                      0,                                                                                                                                                                                                                                                                                                                                                                                                                                                                                                                                                                                                                    0,                                                                                                                                                                                                                                                                                                                                                                                                                                                                                                                                                                                                                    0,                                                                                                                                                                                                                                                                                                                                                                                                                                                                                                                                                                                                                    0,                                                                                                                                                                                                                                                                                                                                                                                                                                                                                                                      0,                                                                                                                                                                                                                                                                                                                                                                                                                                                                                                                      0,                                                                                                                                                                                                                                                                                                                                                                                                                                                                                                                      0,           0,           0,           0, 0, 0, 0,    0,    0,    1,      0,      0,   1/50,                                 0,                                 0,                                 0;
                                                                                                                                                                                                                                                                                                                                                                                                                                                                                                                                                              2*q4*(xa_y - ya2) - 2*q1*(xa_x - ya1) - 2*q3*(xa_z - ya3),                                                                                                                                                                                                                                                                                                                                                                                                                                                                                                                                                          - 2*q2*(xa_x - ya1) - 2*q3*(xa_y - ya2) - 2*q4*(xa_z - ya3),                                                                                                                                                                                                                                                                                                                                                                                                                                                                                                                                                            2*q3*(xa_x - ya1) - 2*q2*(xa_y - ya2) - 2*q1*(xa_z - ya3),                                                                                                                                                                                                                                                                                                                                                                                                                                                                                                                                                            2*q1*(xa_y - ya2) + 2*q4*(xa_x - ya1) - 2*q2*(xa_z - ya3),                                                                                                                                                                                                                                                                                                                                                                                                                                                                                                                      0,                                                                                                                                                                                                                                                                                                                                                                                                                                                                                                                      0,                                                                                                                                                                                                                                                                                                                                                                                                                                                                                                                      0,           0,           0,           0, 0, 0, 0,    0,    0,    0,      0,      0,      0,       - q1^2 - q2^2 + q3^2 + q4^2,                 2*q1*q4 - 2*q2*q3,               - 2*q1*q3 - 2*q2*q4;
                                                                                                                                                                                                                                                                                                                                                                                                                                                                                                                                                              2*q2*(xa_z - ya3) - 2*q4*(xa_x - ya1) - 2*q1*(xa_y - ya2),                                                                                                                                                                                                                                                                                                                                                                                                                                                                                                                                                            2*q2*(xa_y - ya2) - 2*q3*(xa_x - ya1) + 2*q1*(xa_z - ya3),                                                                                                                                                                                                                                                                                                                                                                                                                                                                                                                                                          - 2*q2*(xa_x - ya1) - 2*q3*(xa_y - ya2) - 2*q4*(xa_z - ya3),                                                                                                                                                                                                                                                                                                                                                                                                                                                                                                                                                            2*q4*(xa_y - ya2) - 2*q1*(xa_x - ya1) - 2*q3*(xa_z - ya3),                                                                                                                                                                                                                                                                                                                                                                                                                                                                                                                      0,                                                                                                                                                                                                                                                                                                                                                                                                                                                                                                                      0,                                                                                                                                                                                                                                                                                                                                                                                                                                                                                                                      0,           0,           0,           0, 0, 0, 0,    0,    0,    0,      0,      0,      0,               - 2*q1*q4 - 2*q2*q3,       - q1^2 + q2^2 - q3^2 + q4^2,                 2*q1*q2 - 2*q3*q4;
                                                                                                                                                                                                                                                                                                                                                                                                                                                                                                                                                              2*q3*(xa_x - ya1) - 2*q2*(xa_y - ya2) - 2*q1*(xa_z - ya3),                                                                                                                                                                                                                                                                                                                                                                                                                                                                                                                                                            2*q2*(xa_z - ya3) - 2*q4*(xa_x - ya1) - 2*q1*(xa_y - ya2),                                                                                                                                                                                                                                                                                                                                                                                                                                                                                                                                                            2*q1*(xa_x - ya1) - 2*q4*(xa_y - ya2) + 2*q3*(xa_z - ya3),                                                                                                                                                                                                                                                                                                                                                                                                                                                                                                                                                          - 2*q2*(xa_x - ya1) - 2*q3*(xa_y - ya2) - 2*q4*(xa_z - ya3),                                                                                                                                                                                                                                                                                                                                                                                                                                                                                                                      0,                                                                                                                                                                                                                                                                                                                                                                                                                                                                                                                      0,                                                                                                                                                                                                                                                                                                                                                                                                                                                                                                                      0,           0,           0,           0, 0, 0, 0,    0,    0,    0,      0,      0,      0,                 2*q1*q3 - 2*q2*q4,               - 2*q1*q2 - 2*q3*q4,       - q1^2 + q2^2 + q3^2 - q4^2;
                                                                                                                                                                                                                                                                                                                                                                                                                                                                                                                                                                                                                      0,                                                                                                                                                                                                                                                                                                                                                                                                                                                                                                                                                                                                                    0,                                                                                                                                                                                                                                                                                                                                                                                                                                                                                                                                                                                                                    0,                                                                                                                                                                                                                                                                                                                                                                                                                                                                                                                                                                                                                    0,                                                                                                                                                                                                                                                                                                                                                                                                                                                                                                                      0,                                                                                                                                                                                                                                                                                                                                                                                                                                                                                                                      0,                                                                                                                                                                                                                                                                                                                                                                                                                                                                                                                      0,           0,           0,           0, 0, 0, 0,    0,    0,    0,      0,      0,      0, 9007181240342483/9007199254740992,                                 0,                                 0;
                                                                                                                                                                                                                                                                                                                                                                                                                                                                                                                                                                                                                      0,                                                                                                                                                                                                                                                                                                                                                                                                                                                                                                                                                                                                                    0,                                                                                                                                                                                                                                                                                                                                                                                                                                                                                                                                                                                                                    0,                                                                                                                                                                                                                                                                                                                                                                                                                                                                                                                                                                                                                    0,                                                                                                                                                                                                                                                                                                                                                                                                                                                                                                                      0,                                                                                                                                                                                                                                                                                                                                                                                                                                                                                                                      0,                                                                                                                                                                                                                                                                                                                                                                                                                                                                                                                      0,           0,           0,           0, 0, 0, 0,    0,    0,    0,      0,      0,      0,                                 0, 9007181240342483/9007199254740992,                                 0;
                                                                                                                                                                                                                                                                                                                                                                                                                                                                                                                                                                                                                      0,                                                                                                                                                                                                                                                                                                                                                                                                                                                                                                                                                                                                                    0,                                                                                                                                                                                                                                                                                                                                                                                                                                                                                                                                                                                                                    0,                                                                                                                                                                                                                                                                                                                                                                                                                                                                                                                                                                                                                    0,                                                                                                                                                                                                                                                                                                                                                                                                                                                                                                                      0,                                                                                                                                                                                                                                                                                                                                                                                                                                                                                                                      0,                                                                                                                                                                                                                                                                                                                                                                                                                                                                                                                      0,           0,           0,           0, 0, 0, 0,    0,    0,    0,      0,      0,      0,                                 0,                                 0, 9007181240342483/9007199254740992];
end

function Fu = calcolo_Fu(q1,q2,q3,q4)
Fu =[0, 0, 0, 0, 0, 0,                         0,                         0,                         0, 0, 0, 0;
     0, 0, 0, 0, 0, 0,                         0,                         0,                         0, 0, 0, 0;
     0, 0, 0, 0, 0, 0,                         0,                         0,                         0, 0, 0, 0;
     0, 0, 0, 0, 0, 0,                         0,                         0,                         0, 0, 0, 0;
     1, 0, 0, 0, 0, 0,                         0,                         0,                         0, 0, 0, 0;
     0, 1, 0, 0, 0, 0,                         0,                         0,                         0, 0, 0, 0;
     0, 0, 1, 0, 0, 0,                         0,                         0,                         0, 0, 0, 0;
     0, 0, 0, 1, 0, 0,                         0,                         0,                         0, 0, 0, 0;
     0, 0, 0, 0, 1, 0,                         0,                         0,                         0, 0, 0, 0;
     0, 0, 0, 0, 0, 1,                         0,                         0,                         0, 0, 0, 0;
     0, 0, 0, 0, 0, 0,                         0,                         0,                         0, 0, 0, 0;
     0, 0, 0, 0, 0, 0,                         0,                         0,                         0, 0, 0, 0;
     0, 0, 0, 0, 0, 0,                         0,                         0,                         0, 0, 0, 0;
     0, 0, 0, 0, 0, 0,                         0,                         0,                         0, 0, 0, 0;
     0, 0, 0, 0, 0, 0,                         0,                         0,                         0, 0, 0, 0;
     0, 0, 0, 0, 0, 0,                         0,                         0,                         0, 0, 0, 0;
     0, 0, 0, 0, 0, 0, q1^2 + q2^2 - q3^2 - q4^2,         2*q2*q3 - 2*q1*q4,         2*q1*q3 + 2*q2*q4, 0, 0, 0;
     0, 0, 0, 0, 0, 0,         2*q1*q4 + 2*q2*q3, q1^2 - q2^2 + q3^2 - q4^2,         2*q3*q4 - 2*q1*q2, 0, 0, 0;
     0, 0, 0, 0, 0, 0,         2*q2*q4 - 2*q1*q3,         2*q1*q2 + 2*q3*q4, q1^2 - q2^2 - q3^2 + q4^2, 0, 0, 0;
     0, 0, 0, 0, 0, 0,                         0,                         0,                         0, 1, 0, 0;
     0, 0, 0, 0, 0, 0,                         0,                         0,                         0, 0, 1, 0;
     0, 0, 0, 0, 0, 0,                         0,                         0,                         0, 0, 0, 1];
end

%% %%%%%%%%%%%%%%%%%%%%%%%%%%%%%%%%%%%%%%%%%%%%%%%%%%%%%%%%%%%%%%%%%%%%%%%
     %%%%%%%%% Direct EKF for 6D Pose,  Marco Borraccino %%%%%%%%%%
     %%%%%%%%%   SGN Project, University of Pisa, 2021   %%%%%%%%%%
%%%%%%%%%%%%%%%%%%%%%%%%%%%%%%%%%%%%%%%%%%%%%%%%%%%%%%%%%%%%%%%%%%%%%%%%%%
